simulink library "actuator_control_bus"  (R2018b)
settings: Solver=VariableStepAuto  StartTime=0.0  StopTime=10.0  RelTol=1e-3
undefined symbols (not defined in the file): mtq_dipole_body_Am2, rwa_torque_body_Nm
settings Model: Creator=taylorreynolds  LastModifiedBy=taylorreynolds

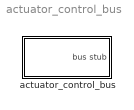
== system actuator_control_bus ==
  actuator_control_bus : Subsystem

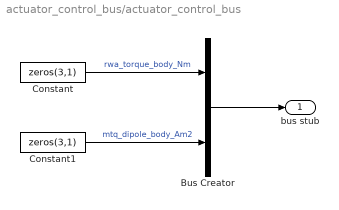
== system actuator_control_bus/actuator_control_bus ==
  Bus Creator : BusCreator  Inputs=rwa_torque_body_Nm,mtq_dipole_body_Am2  OutDataTypeStr=Bus: actuator_control
  Constant : Constant  Value=zeros(3,1)
  Constant1 : Constant  Value=zeros(3,1)
  bus stub : Outport
  wires:
  Bus Creator/1 -> bus stub/1
  Constant/1 -> Bus Creator/1  "rwa_torque_body_Nm"
  Constant1/1 -> Bus Creator/2  "mtq_dipole_body_Am2"
